simulink model "sys_model"  (R2020b)
settings: Solver=VariableStepAuto  StartTime=0.0  StopTime=5  RelTol=1e-3
libraries: simulink x1
settings Model: Creator=Admin  LastModifiedBy=Admin

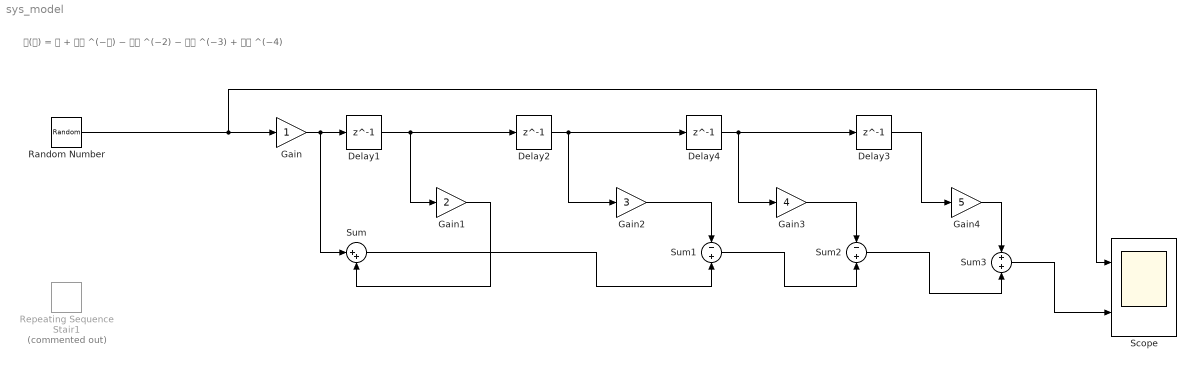
== system sys_model ==
  note: 𝐇(𝐳) = 𝟏 + 𝟐𝐳 ^(−𝟏) − 𝟑𝐳 ^(−2) − 𝟒𝐳 ^(−3) + 𝟓𝐳 ^(−4)
  Delay{1..4} (4 alike) : Delay  DelayLength=1  InitialCondition=0
  Gain : Gain
  Gain1 : Gain  Gain=2
  Gain2 : Gain  Gain=3
  Gain3 : Gain  Gain=4
  Gain4 : Gain  Gain=5
  Random Number : RandomNumber  SampleTime=0.1
  Repeating Sequence Stair1 : simulink/Sources/Repeating Sequence Stair  Commented=on  OutValues=[0 1 0].'  tsamp=-1  OutMin=[]  OutMax=[]  OutDataTypeStr=double  OutputDataTypeScalingMode=double  OutDataType=fixdt(0,8)  ConRadixGroup=Best Precision: Vector-wise  OutScaling=2^-12
  Scope : Scope  NumInputPorts=2
  Sum : Sum  Inputs=|++
  Sum1 : Sum  Inputs=-+
  Sum2 : Sum  Inputs=-+
  Sum3 : Sum
  wires:
  Delay1/1 -> Gain1/1, Delay2/1
  Delay2/1 -> Gain2/1, Delay4/1
  Delay4/1 -> Gain3/1, Delay3/1
  Delay3/1 -> Gain4/1
  Random Number/1 -> Scope/1, Gain/1
  Sum3/1 -> Scope/2
  Gain/1 -> Sum/1, Delay1/1
  Gain1/1 -> Sum/2
  Gain2/1 -> Sum1/1
  Sum/1 -> Sum1/2
  Sum1/1 -> Sum2/2
  Gain3/1 -> Sum2/1
  Sum2/1 -> Sum3/2
  Gain4/1 -> Sum3/1
